simulink model "Setup_for_simulations"  (R2019a)
settings: Solver=VariableStepAuto  StartTime=0.0  StopTime=10.0  RelTol=1e-3
values from neighbouring files (symbols this model uses):
  A = [0, 1, 0; m22*m0/(m11*m22-m12*m21), 0, 0; -m21*m0/(m11*m22-m12*m21), 0, 0]    [Inverted_Pendulum_Simulations.m]
  B = [0; -m12*Km/(m11*m22-m12*m21); m11*Km/(m11*m22-m12*m21)]    [Inverted_Pendulum_Simulations.m]
  C = eye(3)    [Inverted_Pendulum_Simulations.m]
  Imax = 5.6    [Inverted_Pendulum_Simulations.m]
  Iw = 9.189*10^-4    (= 0.0009189)    [Inverted_Pendulum_Simulations.m]
  K_lqr = lqr(A, B, Q, R)    [Inverted_Pendulum_Simulations.m]
libraries: simulink x4
settings Model: Creator=DF_Local  LastModifiedBy=DF_Local

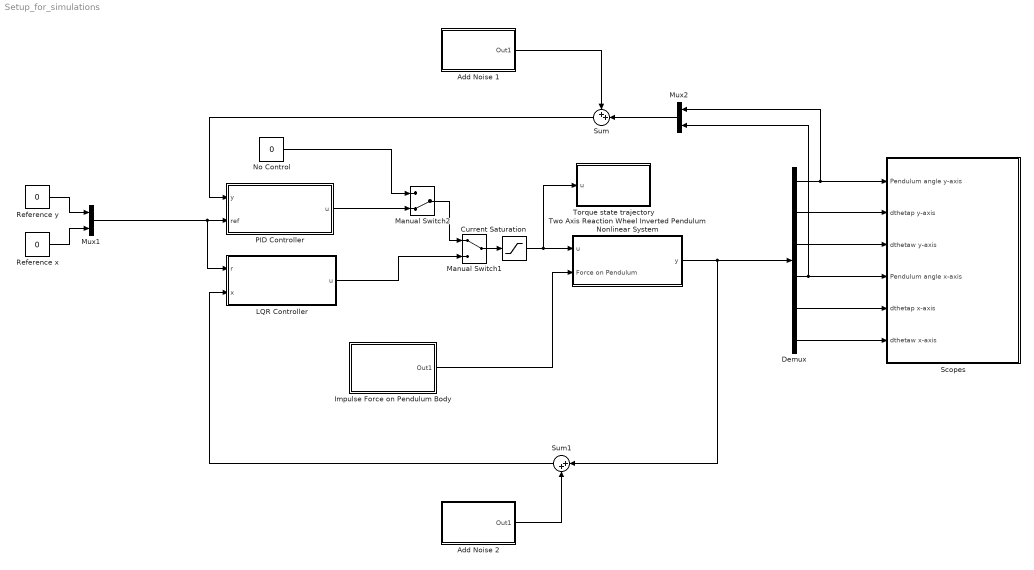
== system Setup_for_simulations ==
  Add Noise 1 : Subsystem
  Add Noise 2 : Subsystem
  Current Saturation : Saturate  UpperLimit=Imax  LowerLimit=-Imax
  Demux : Demux  Outputs=6
  Impulse Force on Pendulum Body : Subsystem
  LQR Controller : Subsystem
  Manual Switch1 : ManualSwitch
  Manual Switch2 : ManualSwitch  CurrentSetting=0
  Mux1 : Mux  Inputs=2
  Mux2 : Mux  Inputs=2
  No Control : Constant  Value=0
  PID Controller : Subsystem
  Reference x : Constant  Value=0
  Reference y : Constant  Value=0
  Scopes : Subsystem
  Sum : Sum  Inputs=++|
  Sum1 : Sum  Inputs=|++
  Torque state trajectory : Subsystem
  Two Axis Reaction Wheel Inverted Pendulum Nonlinear System : Subsystem
  wires:
  Two Axis Reaction Wheel Inverted Pendulum Nonlinear System/1(y) -> Sum1/1, Demux/1
  Mux2/1 -> Sum/2
  Sum1/1 -> LQR Controller/2(x)
  Reference y/1 -> Mux1/1
  Current Saturation/1 -> Torque state trajectory/1(u), Two Axis Reaction Wheel Inverted Pendulum Nonlinear System/1(u)
  No Control/1 -> Manual Switch2/1
  Sum/1 -> PID Controller/1(y)
  Manual Switch1/1 -> Current Saturation/1
  Mux1/1 -> LQR Controller/1(r), PID Controller/2(ref)
  PID Controller/1(u) -> Manual Switch2/2
  Reference x/1 -> Mux1/2
  Demux/4 -> Mux2/2, Scopes/4(Pendulum angle x-axis)
  LQR Controller/1(u) -> Manual Switch1/2
  Demux/1 -> Scopes/1(Pendulum angle y-axis), Mux2/1
  Manual Switch2/1 -> Manual Switch1/1
  Demux/2 -> Scopes/2(dthetap y-axis)
  Demux/3 -> Scopes/3(dthetaw y-axis)
  Demux/5 -> Scopes/5(dthetap x-axis)
  Demux/6 -> Scopes/6(dthetaw x-axis)
  Add Noise 1/1(Out1) -> Sum/1
  Add Noise 2/1(Out1) -> Sum1/2
  Impulse Force on Pendulum Body/1(Out1) -> Two Axis Reaction Wheel Inverted Pendulum Nonlinear System/2(Force on Pendulum)

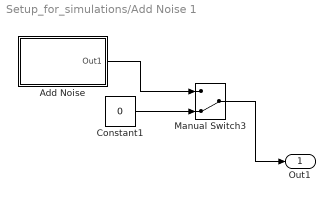
== system Setup_for_simulations/Add Noise 1 ==
  Add Noise : Subsystem
  Constant1 : Constant  Value=0
  Manual Switch3 : ManualSwitch  CurrentSetting=0
  Out1 : Outport
  wires:
  Constant1/1 -> Manual Switch3/2
  Manual Switch3/1 -> Out1/1
  Add Noise/1(Out1) -> Manual Switch3/1

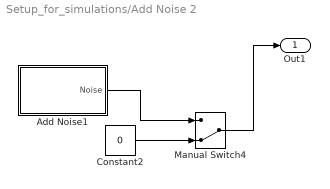
== system Setup_for_simulations/Add Noise 2 ==
  Add Noise1 : Subsystem
  Constant2 : Constant  Value=0
  Manual Switch4 : ManualSwitch  CurrentSetting=0
  Out1 : Outport
  wires:
  Constant2/1 -> Manual Switch4/2
  Add Noise1/1(Noise) -> Manual Switch4/1
  Manual Switch4/1 -> Out1/1

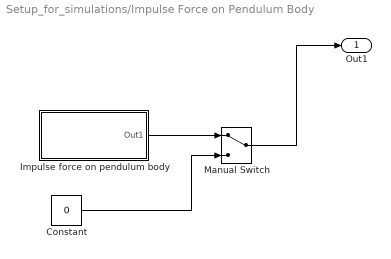
== system Setup_for_simulations/Impulse Force on Pendulum Body ==
  Constant : Constant  Value=0
  Impulse force on pendulum body : Subsystem
  Manual Switch : ManualSwitch
  Out1 : Outport
  wires:
  Constant/1 -> Manual Switch/2
  Manual Switch/1 -> Out1/1
  Impulse force on pendulum body/1(Out1) -> Manual Switch/1

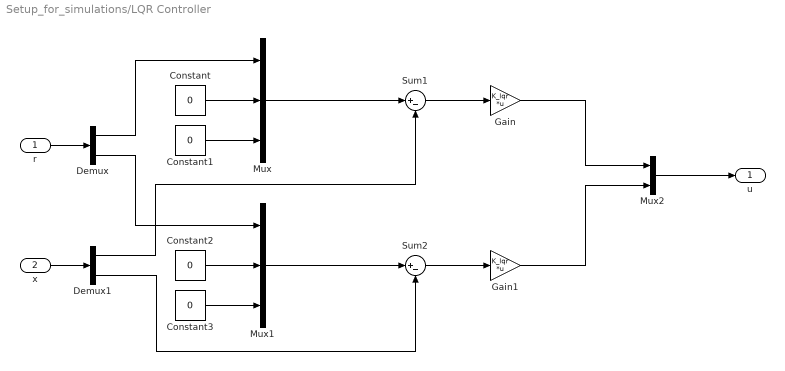
== system Setup_for_simulations/LQR Controller ==
  r : Inport
  x : Inport  Port=2
  Constant{,1..3} (4 alike) : Constant  Value=0
  Demux : Demux  Outputs=2
  Demux1 : Demux  Outputs=2
  Gain : Gain  Gain=K_lqr  Multiplication=Matrix(K*u)
  Gain1 : Gain  Gain=K_lqr  Multiplication=Matrix(K*u)
  Mux : Mux  Inputs=3
  Mux1 : Mux  Inputs=3
  Mux2 : Mux  Inputs=2
  Sum1 : Sum  Inputs=|+-
  Sum2 : Sum  Inputs=|+-
  u : Outport
  wires:
  Sum1/1 -> Gain/1
  Gain/1 -> Mux2/1
  Constant/1 -> Mux/2
  Constant1/1 -> Mux/3
  Mux/1 -> Sum1/1
  Constant3/1 -> Mux1/3
  Mux1/1 -> Sum2/1
  Demux1/2 -> Sum2/2
  Demux/2 -> Mux1/1
  Gain1/1 -> Mux2/2
  Constant2/1 -> Mux1/2
  Sum2/1 -> Gain1/1
  r/1 -> Demux/1
  Demux/1 -> Mux/1
  x/1 -> Demux1/1
  Demux1/1 -> Sum1/2
  Mux2/1 -> u/1

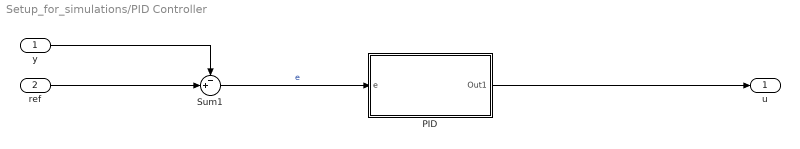
== system Setup_for_simulations/PID Controller ==
  y : Inport
  ref : Inport  Port=2
  PID : Subsystem
  Sum1 : Sum  Inputs=-+|
  u : Outport
  wires:
  ref/1 -> Sum1/2
  y/1 -> Sum1/1
  Sum1/1 -> PID/1(e)  "e"
  PID/1(Out1) -> u/1

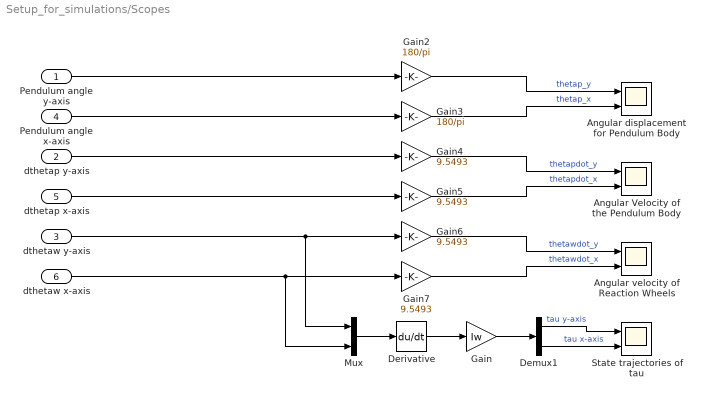
== system Setup_for_simulations/Scopes ==
  Pendulum angle y-axis : Inport
  dthetap y-axis : Inport  Port=2
  dthetaw y-axis : Inport  Port=3
  Pendulum angle x-axis : Inport  Port=4
  dthetap x-axis : Inport  Port=5
  dthetaw x-axis : Inport  Port=6
  Angular Velocity of the Pendulum Body : Scope  NumInputPorts=2
  Angular displacement for Pendulum Body : Scope  NumInputPorts=2
  Angular velocity of Reaction Wheels : Scope  NumInputPorts=2
  Demux1 : Demux  Outputs=2
  Derivative : Derivative
  Gain : Gain  Gain=Iw
  Gain2 : Gain  Gain=180/pi
  Gain3 : Gain  Gain=180/pi
  Gain{4..7} (4 alike) : Gain  Gain=9.5493
  Mux : Mux  Inputs=2
  State trajectories of tau : Scope  NumInputPorts=2
  wires:
  Gain/1 -> Demux1/1
  Mux/1 -> Derivative/1
  dthetaw y-axis/1 -> Mux/1, Gain6/1
  dthetaw x-axis/1 -> Mux/2, Gain7/1
  Gain4/1 -> Angular Velocity of the Pendulum Body/1  "thetapdot_y"
  Demux1/2 -> State trajectories of tau/2  "tau x-axis"
  Derivative/1 -> Gain/1
  Gain7/1 -> Angular velocity of Reaction Wheels/2  "thetawdot_x"
  Gain6/1 -> Angular velocity of Reaction Wheels/1  "thetawdot_y"
  Gain3/1 -> Angular displacement for Pendulum Body/2  "thetap_x"
  Gain2/1 -> Angular displacement for Pendulum Body/1  "thetap_y"
  Gain5/1 -> Angular Velocity of the Pendulum Body/2  "thetapdot_x"
  Demux1/1 -> State trajectories of tau/1  "tau y-axis"
  Pendulum angle y-axis/1 -> Gain2/1
  Pendulum angle x-axis/1 -> Gain3/1
  dthetap y-axis/1 -> Gain4/1
  dthetap x-axis/1 -> Gain5/1

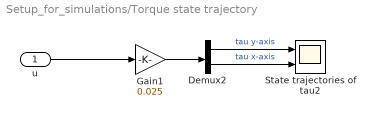
== system Setup_for_simulations/Torque state trajectory ==
  u : Inport
  Demux2 : Demux  Outputs=2
  Gain1 : Gain  Gain=0.025
  State trajectories of tau2 : Scope  NumInputPorts=2
  wires:
  Gain1/1 -> Demux2/1
  Demux2/2 -> State trajectories of tau2/2  "tau x-axis"
  Demux2/1 -> State trajectories of tau2/1  "tau y-axis"
  u/1 -> Gain1/1

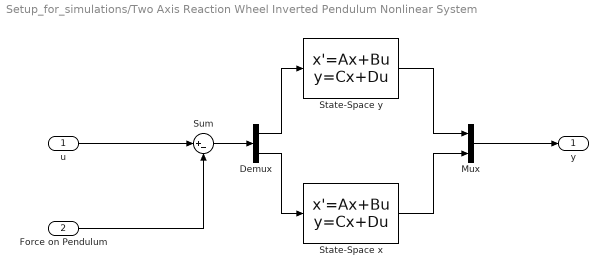
== system Setup_for_simulations/Two Axis Reaction Wheel Inverted Pendulum Nonlinear System ==
  u : Inport
  Force on Pendulum : Inport  Port=2
  Demux : Demux  Outputs=2
  Mux : Mux  Inputs=2
  State-Space x : StateSpace  A=A  B=B  C=C  D=[0; 0; 0]  InitialCondition=[-pi/30; 0; 0]
  State-Space y : StateSpace  A=A  B=B  C=C  D=[0; 0; 0]  InitialCondition=[pi/30; 0; 0]
  Sum : Sum  Inputs=|+-
  y : Outport
  wires:
  Force on Pendulum/1 -> Sum/2
  u/1 -> Sum/1
  State-Space y/1 -> Mux/1
  State-Space x/1 -> Mux/2
  Demux/2 -> State-Space x/1
  Sum/1 -> Demux/1
  Demux/1 -> State-Space y/1
  Mux/1 -> y/1

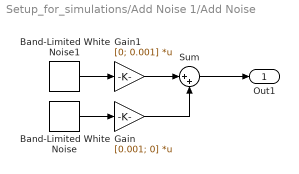
== system Setup_for_simulations/Add Noise 1/Add Noise ==
  Band-Limited White Noise : simulink/Sources/Band-Limited White Noise  Cov=[0.1]  Ts=0.01  seed=[23341]
  Band-Limited White Noise1 : simulink/Sources/Band-Limited White Noise  Cov=[0.1]  Ts=0.01  seed=[23340]
  Gain : Gain  Gain=[0.001; 0]  Multiplication=Matrix(K*u)
  Gain1 : Gain  Gain=[0; 0.001]  Multiplication=Matrix(K*u)
  Sum : Sum  Inputs=|++
  Out1 : Outport
  wires:
  Band-Limited White Noise1/1 -> Gain1/1
  Sum/1 -> Out1/1
  Band-Limited White Noise/1 -> Gain/1
  Gain1/1 -> Sum/1
  Gain/1 -> Sum/2

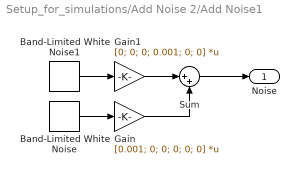
== system Setup_for_simulations/Add Noise 2/Add Noise1 ==
  Band-Limited White Noise : simulink/Sources/Band-Limited White Noise  Cov=[0.1]  Ts=0.01  seed=[23341]
  Band-Limited White Noise1 : simulink/Sources/Band-Limited White Noise  Cov=[0.1]  Ts=0.01  seed=[23340]
  Gain : Gain  Gain=[0.001; 0; 0; 0; 0; 0]  Multiplication=Matrix(K*u)
  Gain1 : Gain  Gain=[0; 0; 0; 0.001; 0; 0]  Multiplication=Matrix(K*u)
  Sum : Sum  Inputs=|++
  Noise : Outport
  wires:
  Band-Limited White Noise1/1 -> Gain1/1
  Sum/1 -> Noise/1
  Band-Limited White Noise/1 -> Gain/1
  Gain1/1 -> Sum/1
  Gain/1 -> Sum/2

== system Setup_for_simulations/Impulse Force on Pendulum Body/Impulse force on pendulum body ==
  Mux4 : Mux  Inputs=2
  Pulse Generator1 : DiscretePulseGenerator  PulseType=Time based  Amplitude=-100  Period=10  PulseWidth=0.3  PhaseDelay=5
  Pulse Generator2 : DiscretePulseGenerator  PulseType=Time based  Amplitude=200  Period=10  PulseWidth=0.3  PhaseDelay=5
  Out1 : Outport
  wires:
  Pulse Generator2/1 -> Mux4/1
  Pulse Generator1/1 -> Mux4/2
  Mux4/1 -> Out1/1

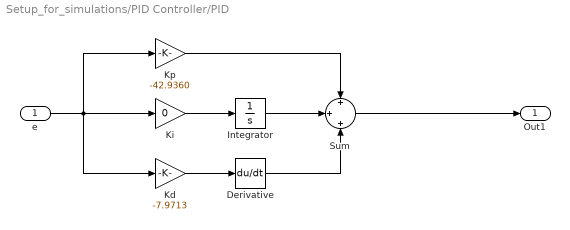
== system Setup_for_simulations/PID Controller/PID ==
  e : Inport
  Derivative : Derivative
  Integrator : Integrator
  Kd : Gain  Gain=-7.9713
  Ki : Gain  Gain=0
  Kp : Gain  Gain=-42.9360
  Sum : Sum  Inputs=+|+|+
  Out1 : Outport
  wires:
  e/1 -> Kp/1, Kd/1, Ki/1
  Sum/1 -> Out1/1
  Integrator/1 -> Sum/2
  Kd/1 -> Derivative/1
  Ki/1 -> Integrator/1
  Derivative/1 -> Sum/3
  Kp/1 -> Sum/1
